simulink library "lib_sig_fault_tolerate"  (R2020a)
settings: Solver=VariableStepAuto  StartTime=0.0  StopTime=10.0  RelTol=1e-3
settings Model: Creator=Administrator  LastModifiedBy=Administrator

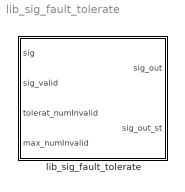
== system lib_sig_fault_tolerate ==
  lib_sig_fault_tolerate : Stateflow chart  TreatAsAtomicUnit=on

== stateflow chart lib_sig_fault_tolerate/lib_sig_fault_tolerate ==
  state good
    en:
    sig_out_st = Good;
    cal_sig_out();
    du:
    cal_sig_out();
  state shaky
    en:
    sig_out_st = Shaky;
    acum_numInvalid = 2;
    cal_sig_out();
    du:
    cal_sig_out();  count_numInvalid();
  state bad
    en:
    sig_out_st = Bad;
    acum_numInvalid =  max_numInvalid;
    cal_sig_out();
    du:
    cal_sig_out();  count_numInvalid();
  bad -> good [order 2] : [acum_numInvalid <= 0 ]
  good -> shaky : [ ~sig_valid ]
  shaky -> good [order 2] : [acum_numInvalid <= 0]
  shaky -> bad [order 1] : [acum_numInvalid >= 2*tolerat_numInvalid ]
  bad -> bad [order 1] : [ ~sig_valid ]
  (default) -> bad : {sig_out_old = 0; }
  data: sig input single; sig_out output single; sig_valid input boolean; sig_out_st output Enum: Enum_sig_status; sig_out_old local single; tolerat_numInvalid input int8; acum_numInvalid local int8; max_numInvalid input int8
  function cal_sig_out:
    | function cal_sig_out
    | 
    | if ( ~sig_valid )
    |     sig_out = sig_out_old;
    | 
    | else        % valid
    | 
    |     sig_out = sig; 
    |     
    | end
    | 
    | 
    | sig_out_old = sig_out;
  function count_numInvalid:
    | function count_numInvalid
    | 
    | 
    | if ( ~sig_valid )
    |     acum_numInvalid = acum_numInvalid + 2;
    |     if acum_numInvalid > max_numInvalid
    |         acum_numInvalid = max_numInvalid;
    |     end       
    | else
    |     acum_numInvalid = acum_numInvalid - 1;
    |     if acum_numInvalid < 0
    |         acum_numInvalid = int8(0);
    |     end
    | end
